simulink model "lab2B"  (R2024a)
settings: Solver=VariableStepAuto  StartTime=0.0  StopTime=10.0  RelTol=1e-3
settings Model: Creator=pktubs  LastModifiedBy=pktubs

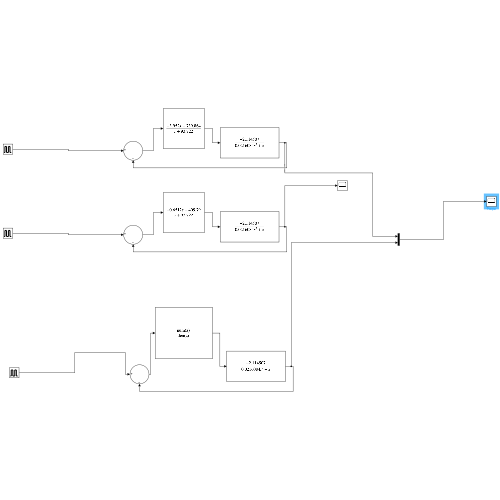
[thumbnail: Simulink's stored preview of the top-level diagram]
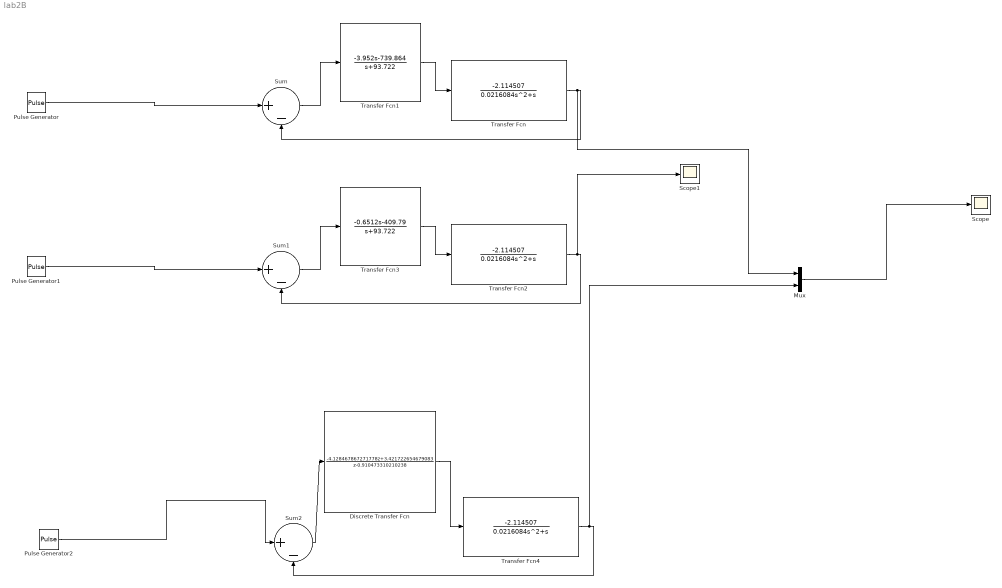
== system lab2B ==
  Discrete Transfer Fcn : DiscreteTransferFcn  Numerator=[-4.128467867271778 3.421722654679083]  Denominator=[1 -0.910473310210238]  SampleTime=0.001
  Mux : Mux  Inputs=2
  Pulse Generator : DiscretePulseGenerator  PulseType=Time based  Amplitude=1.4  PulseWidth=50
  Pulse Generator1 : DiscretePulseGenerator  PulseType=Time based  Amplitude=1.4  PulseWidth=50
  Pulse Generator2 : DiscretePulseGenerator  PulseType=Time based  Amplitude=1.4  PulseWidth=50
  Scope : Scope
  Scope1 : Scope
  Sum : Sum  Inputs=|+-
  Sum1 : Sum  Inputs=|+-
  Sum2 : Sum  Inputs=|+-
  Transfer Fcn : TransferFcn  Numerator=[-2.114507]  Denominator=[0.0216084 1 0]
  Transfer Fcn1 : TransferFcn  Numerator=[-3.952 -739.864]  Denominator=[1 93.722]
  Transfer Fcn2 : TransferFcn  Numerator=[-2.114507]  Denominator=[0.0216084 1 0]
  Transfer Fcn3 : TransferFcn  Numerator=[-0.6512 -409.79]  Denominator=[1 93.722]
  Transfer Fcn4 : TransferFcn  Numerator=[-2.114507]  Denominator=[0.0216084 1 0]
  wires:
  Pulse Generator/1 -> Sum/1
  Sum/1 -> Transfer Fcn1/1
  Transfer Fcn1/1 -> Transfer Fcn/1
  Transfer Fcn/1 -> Mux/1, Sum/2
  Transfer Fcn2/1 -> Scope1/1, Sum1/2
  Sum1/1 -> Transfer Fcn3/1
  Transfer Fcn3/1 -> Transfer Fcn2/1
  Pulse Generator1/1 -> Sum1/1
  Transfer Fcn4/1 -> Mux/2, Sum2/2
  Sum2/1 -> Discrete Transfer Fcn/1
  Discrete Transfer Fcn/1 -> Transfer Fcn4/1
  Pulse Generator2/1 -> Sum2/1
  Mux/1 -> Scope/1
